simulink model "lqr_inner"  (R2017a)
settings: Solver=ode5  StartTime=0.0  StopTime=50  FixedStep=Ts  RelTol=1e-3  EnableMultiTasking=on
values from neighbouring files (symbols this model uses):
  Ki_lqr = [8.66025403784  0  0; 0  0.1  0; 0  0  0.1]    [K_lqr.mat]    (also in lqr_inner_synthesis.m = -K(:,7:end))
  Kx_lqr = [13.6588017709 0 0 7.88446073405 0 0 0 0.182798226623 0 0 0 0.193348614018 ... (18 elements, 3x6)]    [K_lqr.mat]    (also in lqr_inner_synthesis.m = K(:,1:6))
undefined symbols (not defined in the file or in its folder): B_inner_inv, gra, KT, mass
settings Model: Creator=dtnguyen  LastModifiedBy=ducnguyen
settings DataIOCC: LimitDataPoints=on  SaveFormat=Array
settings OptimizationCC: DefaultParameterBehavior=Inlined  UseFloatMulNetSlope=on  InlineInvariantSignals=on  PassReuseOutputArgsThreshold=0  EfficientFloat2IntCast=on
settings DebuggingCC: ParameterTunabilityLossMsg=error  SFUnexpectedBacktrackingDiag=warning  SFNoUnconditionalDefaultTransitionDiag=warning  SFExecutionAtInitializationDiag=none
settings HardwareCC: ProdBitPerPointer=32  ProdBitPerSizeT=32  ProdBitPerPtrDiffT=32  ProdLargestAtomicFloat=None  ProdIntDivRoundTo=Undefined  ProdEndianess=Unspecified  ProdWordSize=32  ProdHWDeviceType=32-bit Generic
settings ModelReferenceCC: PropagateSignalLabelsOutOfModel=off
settings RTWCC: PackageGeneratedCodeAndArtifacts=on  PackageName=myCodeExport  GenerateReport=on  Toolchain=Catkin  BuildConfiguration=Faster Runs  LaunchReport=on  TargetLang=C++  CheckMdlBeforeBuild=Warning
settings CodeAppCC: ForceParamTrailComments=on  OperatorAnnotations=on  MATLABSourceComments=on
settings GRTTargetCC: TargetLangStandard=C++03 (ISO)  MatFileLogging=off  MultiInstanceERTCode=on  CodeInterfacePackaging=C++ class
settings ConfigComp: CovMetricSettings=dw  CovHtmlReporting=on  CovSaveCumulativeToWorkspaceVar=on  CovSaveSingleToWorkspaceVar=on  CovExternalEMLEnable=off

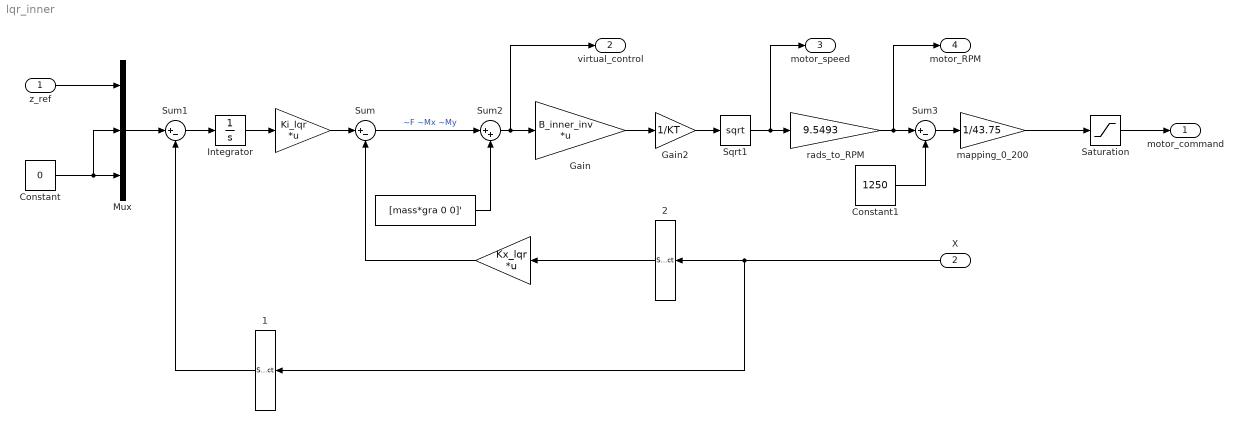
== system lqr_inner ==
  z_ref : Inport  PortDimensions=1
  X : Inport  Port=2  PortDimensions=12
  " " : Gain  Gain=Ki_lqr  Multiplication=Matrix(K*u)
  "              " : Constant  Value=[mass*gra 0 0]'
  "                   " : Gain  Gain=Kx_lqr  Multiplication=Matrix(K*u)
  "                    1" : Selector  InputPortWidth=12  IndexOptions=Index vector (dialog)  Indices=[3 7 8]  OutputSizes=1
  "                    2" : Selector  InputPortWidth=12  IndexOptions=Index vector (dialog)  Indices=[3 6 7 8 10 11]  OutputSizes=1
  Constant : Constant  Value=0
  Constant1 : Constant  Value=1250  VectorParams1D=off  SampleTime=-1
  Gain : Gain  Gain=B_inner_inv  Multiplication=Matrix(K*u)
  Gain2 : Gain  Gain=1/KT
  Integrator : Integrator  InitialCondition=[0 0 0]'
  Mux : Mux  Inputs=3
  Saturation : Saturate  UpperLimit=200  LowerLimit=0
  Sqrt1 : Sqrt  SaturateOnIntegerOverflow=on
  Sum : Sum  Inputs=|+-
  Sum1 : Sum  Inputs=|+-
  Sum2 : Sum  Inputs=|++
  Sum3 : Sum  Inputs=|+-
  mapping_0_200 : Gain  Gain=1/43.75
  rads_to_RPM : Gain  Gain=9.5493
  motor_command : Outport  PortDimensions=6
  virtual_control : Outport  Port=2  PortDimensions=3
  motor_speed : Outport  Port=3  PortDimensions=6
  motor_RPM : Outport  Port=4  PortDimensions=6
  wires:
  Gain2/1 -> Sqrt1/1
  "                    2"/1 -> "                   "/1
  Sum1/1 -> Integrator/1
  " "/1 -> Sum/1
  "                    1"/1 -> Sum1/2
  Integrator/1 -> " "/1
  "                   "/1 -> Sum/2
  Gain/1 -> Gain2/1
  X/1 -> "                    2"/1, "                    1"/1
  z_ref/1 -> Mux/1
  Mux/1 -> Sum1/1
  Sqrt1/1 -> motor_speed/1, rads_to_RPM/1
  Sum2/1 -> virtual_control/1, Gain/1
  Sum/1 -> Sum2/1  "~F ~Mx ~My"
  "              "/1 -> Sum2/2
  Constant/1 -> Mux/2, Mux/3
  Constant1/1 -> Sum3/2
  rads_to_RPM/1 -> Sum3/1, motor_RPM/1
  Sum3/1 -> mapping_0_200/1
  mapping_0_200/1 -> Saturation/1
  Saturation/1 -> motor_command/1
